simulink library "mbd_s32k1xx_ec_toolbox"  (Simulink 9.0)
settings: Solver=FixedStepDiscrete  StartTime=0.0  StopTime=10.0  FixedStep=0.1  RelTol=1e-3  EnableMultiTasking=on
InitFcn:
  | mbd_s32k_consistency_checks(bdroot(gcs));
(part 5 of 8)

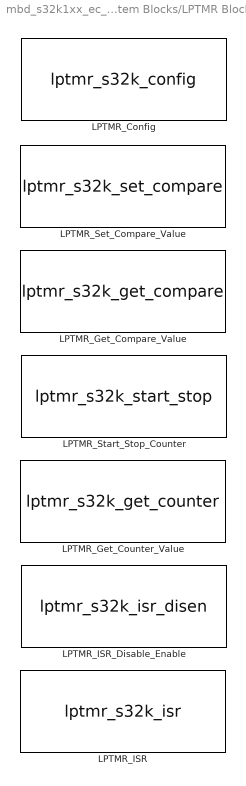
== system mbd_s32k1xx_ec_toolbox/Core and System Blocks/LPTMR Blocks ==
  LPTMR_Config : S-Function  FunctionName=lptmr_s32k_config  SFunctionDeploymentMode=off  EnableBusSupport=off  mask(lptmr_s32k_config){work_mode=Time Counter mode, compare_value=1, compare_value_units=Ticks, pin_select=Count pulses from pin alternative 1, pin_polarity=Count pulse on rising edge, pin_trgmux_source=Trigger MUX input 1, pin_gpio=PTE11: [LPTMR0_ALT1 | Low Power Timer Input Channel], show_adv_opts=on, input_clock=SIRC DIV2 clock, prescaler=Timer mode: prescaler 2, Glitch filter mode: invalid, bypass_prescaler=off, free_run=off, start_counter=on, enable_isr=off}
      mask prompts: work_mode "Mode Select"; compare_value "Compare Value"; compare_value_units "Compare Value Units"; pin_select "Pin Source"; pin_polarity "Pin Polarity"; pin_trgmux_source "TRGMUX Source"; pin_gpio "Input Pin"; show_adv_opts "Show advanced options"; input_clock "Prescaler Clock Select"; prescaler "Prescale Value"; bypass_prescaler "Prescaler Bypass"; free_run "Timer Free-Running Counter"; start_counter "Start  LPTMR counter immediatly after initialization"; enable_isr "Enable ISR immediatly after initialization"
      mask help: This block allows the user to configure the LPTMR module.
      mask init:
      | [maskStr, labels] = mbd_s32k_lptmr_init();
      | 
      | set_param(gcb, 'MaskDisplay', labels);
      settings: NameChangeFcn=mbd_s32k_name_check(gcb);
      mask Help: web(fullfile(mbd_s32k_block_help, 'lptmr', 'lptmr_config.html'));
      mask TypeOptions work_mode: Time Counter mode | Pulse Counter mode
      mask Callback work_mode:
      | mbd_s32k_lptmr_config_cbk('mode')
      | mbd_s32k_lptmr_config_cbk('pin')
      mask TypeOptions compare_value_units: Ticks | Microseconds
      mask Callback compare_value_units: mbd_s32k_lptmr_config_cbk('units')
      mask TypeOptions pin_select: Count pulses from pin alternative 1 | Count pulses from pin alternative 2 | Count pulses from pin alternative 3 | Count pulses from TRGMUX trigger
      mask Callback pin_select:
      | mbd_s32k_lptmr_config_cbk('trgmux');
      | mbd_s32k_lptmr_config_cbk('pin');
      mask TypeOptions pin_polarity: Count pulse on rising edge | Count pulse on falling edge
      mask TypeOptions pin_trgmux_source: Trigger function is disabled | Trigger MUX input 0 | Trigger MUX input 1 | Trigger MUX input 2 | Trigger MUX input 3 | Trigger MUX input 4 | Trigger MUX input 5 | Trigger MUX input 6 | Trigger MUX input 7 | Trigger MUX input 8 | Trigger MUX input 9 | Trigger MUX input 10 | Trigger MUX input 11 | CMP0 Output | LPIT Channel 0 | LPIT Channel 1 | LPIT Channel 2 | LPIT Channel 3 | LPTMR0 Trigger | FTM0 Initialize Trigger | FTM0 External Trigger | FTM1 Initialize Trigger | FTM1 External Trigger | FTM2 Initialize Trigger | FTM2 External Trigger | FTM3 Initialize Trigger | FTM3 External Trigger | ADC0_COCOA | ADC0_COCOB | ADC1_COCOA | ADC1_COCOB | PDB0 Channel 0 Trigger | PDB0 Pulse out | PDB1 Channel 0 Trigger | PDB1 Pulse out | RTC Alarm | RTC Seconds Counter | Flex IO Trigger 0 | Flex IO Trigger 1 | Flex IO Trigger 2 | Flex IO Trigger 3 | LPUART0 RX Data | LPUART0 TX Data | LPUART0 RX Idle | LPUART1 RX Data | LPUART1 TX Data | LPUART1 RX Idle | LPI2C0 Master Stop | LPI2C0 Slave Stop | LPI2C1 Master Stop | LPI2C1 Slave Stop | LPSPI0 Frame | LPSPI0 RX Data | LPSPI1 Frame | LPSPI1 RX Data | SIM Software Trigger
      mask Callback pin_trgmux_source: mbd_s32k_lptmr_config_cbk('pin');
      mask TypeOptions pin_gpio: PTE11: [LPTMR0_ALT1 | Low Power Timer Input Channel]
      mask Callback show_adv_opts: mbd_s32k_lptmr_config_cbk('show_adv_opts')
      mask TypeOptions input_clock: SIRC DIV2 clock | 1kHz LPO clock | RTC clock | PCC configured clock
      mask TypeOptions prescaler: Timer mode: prescaler 2, Glitch filter mode: invalid | Timer mode: prescaler 4, Glitch filter mode: 2 clocks | Timer mode: prescaler 8, Glitch filter mode: 4 clocks | Timer mode: prescaler 16, Glitch filter mode: 8 clocks | Timer mode: prescaler 32, Glitch filter mode: 16 clocks | Timer mode: prescaler 64, Glitch filter mode: 32 clocks | Timer mode: prescaler 128, Glitch filter mode: 64 clocks | Timer mode: prescaler 256, Glitch filter mode: 128 clocks | Timer mode: prescaler 512, Glitch filter mode: 256 clocks | Timer mode: prescaler 1024, Glitch filter mode: 512 clocks | Timer mode: prescaler 2048, Glitch filter mode: 1024 clocks | Timer mode: prescaler 4096, Glitch filter mode: 2048 clocks | Timer mode: prescaler 8192, Glitch filter mode: 4096 clocks | Timer mode: prescaler 16384, Glitch filter mode: 8192 clocks | Timer mode: prescaler 32768, Glitch filter mode: 16384 clocks | Timer mode: prescaler 65536, Glitch filter mode: 32768 clocks
      mask Callback bypass_prescaler: mbd_s32k_lptmr_config_cbk('prescaler')
      mask DialogControl timer_config_group Prompt: Timer configuration
      mask DialogControl source_config_group Prompt: Source configuration
      mask DialogControl prescaler_config_group Prompt: Prescaler configuration
      mask Display:
      | image('nxp_logo.png', 'top-right');
      | disp(maskStr);
  LPTMR_Get_Compare_Value : S-Function  FunctionName=lptmr_s32k_get_compare  Parameters=sFuncParams  SFunctionDeploymentMode=off  EnableBusSupport=off  mask(lptmr_s32k_get_compare){compare_value_units=Ticks}
      mask prompts: compare_value_units "Compare Value Units"
      mask help: This block allows the user to get the compare value in counter tick units or microseconds, for LPTMR.
      mask init:
      | [maskStr, labels, sFuncParams] = mbd_s32k_lptmr_get_compare();
      | 
      | set_param(gcb, 'MaskDisplay', labels);
      settings: NameChangeFcn=mbd_s32k_name_check(gcb);
      mask Help: web(fullfile(mbd_s32k_block_help, 'lptmr', 'lptmr_get_compare.html'));
      mask TypeOptions compare_value_units: Ticks | Microseconds
      mask Display:
      | image('nxp_logo.png', 'top-right');
      | port_label('output', 1, 'Compare Value');
      | disp(maskStr);
  LPTMR_Get_Counter_Value : S-Function  FunctionName=lptmr_s32k_get_counter  SFunctionDeploymentMode=off  EnableBusSupport=off  mask(lptmr_s32k_get_counter){}
      mask help: This block allows the user to get the current counter value in counter ticks units, for LPTMR.
      mask init:
      | [maskStr labels] = mbd_s32k_lptmr_get_counter();
      | 
      | set_param(gcb, 'MaskDisplay', labels);
      settings: NameChangeFcn=mbd_s32k_name_check(gcb);
      mask Help: web(fullfile(mbd_s32k_block_help, 'lptmr', 'lptmr_get_counter.html'));
      mask Display:
      | image('nxp_logo.png', 'top-right');
      | port_label('output', 1, 'Counter Value')
      | disp(maskStr);
  LPTMR_ISR : S-Function  FunctionName=lptmr_s32k_isr  SFunctionDeploymentMode=off  EnableBusSupport=off  mask(lptmr_s32k_isr){}
      mask help: This block allows to call user function on LPTMR interrupt.
      settings: NameChangeFcn=mbd_s32k_name_check(gcb);
      mask Help: web(fullfile(mbd_s32k_block_help, 'lptmr', 'lptmr_isr.html'));
      mask Display:
      | image('nxp_logo.png', 'top-right');
      | disp('LPTMR ISR');
  LPTMR_ISR_Disable_Enable : S-Function  FunctionName=lptmr_s32k_isr_disen  SFunctionDeploymentMode=off  EnableBusSupport=off  mask(lptmr_s32k_isr_disen){set_action=Enable}
      mask prompts: set_action "Action"
      mask help: This block allows the user to enable or disable the LPTMR.
      mask init:
      | [maskStr, labels] = mbd_s32k_lptmr_isr_disen();
      | 
      | set_param(gcb, 'MaskDisplay', labels);
      settings: NameChangeFcn=mbd_s32k_name_check(gcb);
      mask Help: web(fullfile(mbd_s32k_block_help, 'lptmr', 'lptmr_isr_disable_enable.html'));
      mask TypeOptions set_action: Enable | Disable
      mask Display:
      | image('nxp_logo.png', 'top-right');
      | disp(maskStr);
  LPTMR_Set_Compare_Value : S-Function  FunctionName=lptmr_s32k_set_compare  Parameters=sFuncParams  SFunctionDeploymentMode=off  EnableBusSupport=off  mask(lptmr_s32k_set_compare){compare_value_units=Microseconds}
      mask prompts: compare_value_units "Compare Value Units"
      mask help: This block allows the user to set the compare value in counter tick units or microsenconds, for LPTMR.
      mask init:
      | [maskStr, labels, sFuncParams] = mbd_s32k_lptmr_set_compare();
      | 
      | set_param(gcb, 'MaskDisplay', labels);
      settings: NameChangeFcn=mbd_s32k_name_check(gcb);
      mask Help: web(fullfile(mbd_s32k_block_help, 'lptmr', 'lptmr_set_compare.html'));
      mask TypeOptions compare_value_units: Ticks | Microseconds
      mask Display:
      | image('nxp_logo.png', 'top-right');
      | port_label('input', 1, 'Compare Value');
      | disp(maskStr);
  LPTMR_Start_Stop_Counter : S-Function  FunctionName=lptmr_s32k_start_stop  SFunctionDeploymentMode=off  EnableBusSupport=off  mask(lptmr_s32k_start_stop){set_action=Start}
      mask prompts: set_action "Action"
      mask help: This block allows the user to start or stop the LPTMR.
      mask init:
      | [maskStr, labels] = mbd_s32k_lptmr_start_stop();
      | 
      | set_param(gcb, 'MaskDisplay', labels);
      settings: NameChangeFcn=mbd_s32k_name_check(gcb);
      mask Help: web(fullfile(mbd_s32k_block_help, 'lptmr', 'lptmr_start_stop.html'));
      mask TypeOptions set_action: Start | Stop
      mask Display:
      | image('nxp_logo.png', 'top-right');
      | disp(maskStr);

== system mbd_s32k1xx_ec_toolbox/Core and System Blocks/PMC Blocks ==
  PMC_Config : S-Function  FunctionName=pmc_s32k_config  Parameters=sFuncParams  SFunctionDeploymentMode=off  EnableBusSupport=off  mask(pmc_s32k_config){power_mode=Very Low Power Stop (VLPS), sleep_on_exit=off, callback_before=off, callback_after=off, callback_before_after=off, show_adv_opts=off}
      mask prompts: power_mode "Power Mode"; sleep_on_exit "Sleep on exit from ISR"; callback_before "Execute subsystem "Before" entering in selected Power Mode"; callback_after "Execute subsystem "After" exiting from selected Power Mode"; callback_before_after "Execute subsystem "Before and After" selected Power Mode"; show_adv_opts "Show advanced options"
      mask help: This block allows the user to handle the device power modes and trigger subsystems execution at run-time switching between power modes.
      mask init:
      | mbd_s32k_pmc_config_cbk(gcb);
      | 
      | [st,labels] = mbd_s32k_pmc_init(gcb);
      | 
      | set_param(gcb, 'MaskDisplay', labels);
      | 
      | sFuncParams = [callback_before
      |                 callback_after
      |                 callback_before_after]';
      settings: NameChangeFcn=mbd_s32k_name_check(gcb);
      mask Help: web(fullfile(mbd_s32k_block_help, 'pmc', 'pmc_config.html'));
      mask TypeOptions power_mode: Very Low Power Stop (VLPS) | Very Low Power Run (VLPR) | High Speed Run (HSRUN) | Normal Operating (RUN) | Stop System and Bus clocks (STOP1) | Stop System clock and keep Bus clock running (STOP2)
      mask Callback power_mode: mbd_s32k_pmc_config_cbk(gcb);
      mask Callback show_adv_opts: mbd_s32k_pmc_config_cbk(gcb);
      mask DialogControl Control2 Prompt: %<MaskDescription>)
      mask DialogControl container_mode Prompt: General
      mask DialogControl Container20 Prompt: Run/Stop
      mask DialogControl container_callbacks Prompt: Callbacks
      mask Display:
      | image('nxp_logo.png', 'top-right');
      | disp(st);

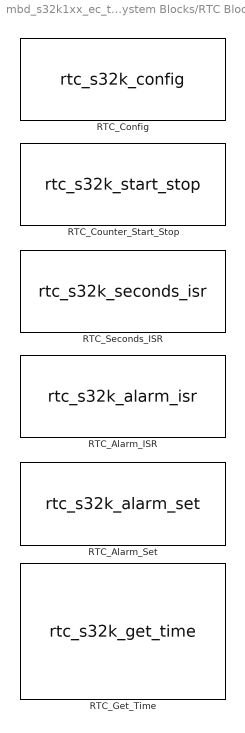
== system mbd_s32k1xx_ec_toolbox/Core and System Blocks/RTC Blocks ==
  RTC_Alarm_ISR : S-Function  FunctionName=rtc_s32k_alarm_isr  SFunctionDeploymentMode=off  EnableBusSupport=off  mask(rtc_s32k_alarm_isr){}
      mask help: This block allows to call user function on RTC interrupt.
      settings: NameChangeFcn=mbd_s32k_name_check(gcb);
      mask Help: web(fullfile(mbd_s32k_block_help, 'rtc', 'rtc_alarm_isr.html'));
      mask Display:
      | image('nxp_logo.png', 'top-right');
      | disp('RTC Alarm ISR');
  RTC_Alarm_Set : S-Function  FunctionName=rtc_s32k_alarm_set  Parameters=sFuncParams  SFunctionDeploymentMode=off  EnableBusSupport=off  mask(rtc_s32k_alarm_set){inputs_enable=on, date_day=1, date_month=1, date_year=1970, time_hour=0, time_min=0, time_sec=0, show_adv_opts=off, repeat=off, interval=0, forever=on, repeats=0}
      mask prompts: inputs_enable "Date/Time as inputs"; date_day "Date (dd/mm/yy)"; time_hour "Time (hh:mm::ss)"; show_adv_opts "Show advanced options"; interval "Repeat interval (seconds)"; forever "Repeat forever"; repeats "Number of repeats"
      mask help: This block allows the user to set an alarm.
      mask init:
      | [st, labels] = mbd_s32k_rtc_alarm_set_init();
      | sFuncParams = [inputs_enable]';
      | set_param(gcb, 'MaskDisplay', labels);
      settings: NameChangeFcn=mbd_s32k_name_check(gcb);
      mask Help: web(fullfile(mbd_s32k_block_help, 'rtc', 'rtc_alarm_set.html'));
      mask Callback inputs_enable: mbd_s32k_rtc_alarm_set_cbk('inputs_enable')
      mask Callback show_adv_opts: mbd_s32k_rtc_alarm_set_cbk('show_adv_opts')
      mask Callback repeat: mbd_s32k_rtc_alarm_set_cbk('repeat_enable')
      mask Callback forever: mbd_s32k_rtc_alarm_set_cbk('repeat_forever')
      mask Display:
      | image('nxp_logo.png', 'top-right');
      | port_label('input', 1, 'Year')
      | port_label('input', 2, 'Month')
      | port_label('input', 3, 'Day')
      | port_label('input', 4, 'Hours')
      | port_label('input', 5, 'Minutes')
      | port_label('input', 6, 'Seconds')
      | disp(st);
  RTC_Config : S-Function  FunctionName=rtc_s32k_config  SFunctionDeploymentMode=off  EnableBusSupport=off  mask(rtc_s32k_config){date_day=1, date_month=1, date_year=1970, time_hour=0, time_min=0, time_sec=0, show_adv_opts=off, clock_input=1KHz LPO, clock_output=Disabled, comp_state=on, comp_value=0, comp_interval=0, state_update=off, state_w_access=off, state_read_only=off, start_counter=on}
      mask prompts: date_day "Date"; time_hour "Time"; show_adv_opts "Show advanced options"; clock_input "Input Clock"; clock_output "Clock Out"; comp_state "Compensation"; comp_value "Compensation value            [-127,128]"; comp_interval "Compensation interval              [0,255]"; state_update "Update"; state_w_access "Non-supervisor write access"; state_read_only "Read-only"; start_counter "Start RTC counter immediatly after initialization"
      mask help: This block allows the user to configure the RTC module.
      mask init:
      | [labels ,maskStr] = mbd_s32k_rtc_config_init();
      | 
      | set_param(gcb, 'MaskDisplay', [labels, newline, 'disp(maskStr);']);
      settings: NameChangeFcn=mbd_s32k_name_check(gcb);
      mask Help: web(fullfile(mbd_s32k_block_help, 'rtc', 'rtc_config.html'));
      mask Callback show_adv_opts: mbd_s32k_rtc_config_cbk('show_adv_opts')
      mask TypeOptions clock_input: 32KHz crystal | 1KHz LPO
      mask TypeOptions clock_output: Disabled | Prescaler output | 32KHz clock
      mask Callback comp_state: mbd_s32k_rtc_config_cbk('compensation')
      mask Callback comp_interval: mbd_s32k_rtc_config_cbk('comp_value')
      mask DialogControl time_config_group Prompt: Time configuration
      mask DialogControl time_config_group_copy Prompt: Time configuration
      mask Display:
      | image('nxp_logo.png', 'top-right');
      | 
      | disp(maskStr);
  RTC_Counter_Start_Stop : S-Function  FunctionName=rtc_s32k_start_stop  SFunctionDeploymentMode=off  EnableBusSupport=off  mask(rtc_s32k_counter_start_stop){set_action=Start}
      mask prompts: set_action "Action"
      mask help: This block allows the user to start or stop the RTC counter.
      mask init:
      | [labels, maskStr] = mbd_s32k_rtc_start_stop();
      | 
      | set_param(gcb, 'MaskDisplay', [labels, 'disp(maskStr);']);
      settings: NameChangeFcn=mbd_s32k_name_check(gcb);
      mask Help: web(fullfile(mbd_s32k_block_help, 'rtc', 'rtc_counter_start_stop.html'));
      mask TypeOptions set_action: Start | Stop
      mask Display:
      | image('nxp_logo.png', 'top-right');
      | disp(maskStr);
  RTC_Get_Time : S-Function  FunctionName=rtc_s32k_get_time  SFunctionDeploymentMode=off  EnableBusSupport=off  mask(rtc_s32k_get_time){}
      mask help: This block returns the time to the user.
      mask init:
      | [st,labels] = mbd_s32k_rtc_get_time_init();
      | set_param(gcb, 'MaskDisplay', labels);
      settings: NameChangeFcn=mbd_s32k_name_check(gcb);
      mask Help: web(fullfile(mbd_s32k_block_help, 'rtc', 'rtc_get_time.html'));
      mask Display:
      | image('nxp_logo.png', 'top-right');
      | port_label('output', 1, 'Year')
      | port_label('output', 2, 'Month')
      | port_label('output', 3, 'Day')
      | port_label('output', 4, 'Hours')
      | port_label('output', 5, 'Minutes')
      | port_label('output', 6, 'Seconds')
      | disp(st);
  RTC_Seconds_ISR : S-Function  FunctionName=rtc_s32k_seconds_isr  SFunctionDeploymentMode=off  EnableBusSupport=off  mask(rtc_s32k_seconds_isr){sec_irq_freq=1Hz}
      mask prompts: sec_irq_freq "Frequency"
      mask help: This block allows to call user function on RTC interrupt.
      mask init:
      | [labels, maskStr] = mbd_s32k_rtc_seconds_isr_init();
      | 
      | set_param(gcb, 'MaskDisplay', [labels, 'disp(maskStr);']);
      settings: NameChangeFcn=mbd_s32k_name_check(gcb);
      mask Help: web(fullfile(mbd_s32k_block_help, 'rtc', 'rtc_seconds_isr.html'));
      mask TypeOptions sec_irq_freq: 1Hz | 2Hz | 4Hz | 8Hz | 16Hz | 32Hz | 64Hz | 128Hz
      mask DialogControl Container3 Prompt: General
      mask Display:
      | image('nxp_logo.png', 'top-right');
      | disp(maskStr);

== system mbd_s32k1xx_ec_toolbox/Core and System Blocks/WDOG Blocks ==
  WDOG_Config : S-Function  FunctionName=wdog_s32k_config  Parameters=sFuncParams  SFunctionDeploymentMode=off  EnableBusSupport=off  mask(wdog_s32k_config){clk_source=LPO clock, window_enable=off, window_value=1000.000, window_value_unit=milliseconds, timeout_value=1000.000, timeout_value_unit=milliseconds, prescaler_enable=on, update_enable=off, int_enable=off, show_adv_opts=off}
      mask prompts: clk_source "Clock source"; window_enable "Window enable"; window_value "Window value"; timeout_value "Timeout value"; prescaler_enable "Prescaler enable"; update_enable "Update enable"; int_enable "Interrupt enable"; show_adv_opts "Show advanced options"
      mask help: This block allows the user to configure the WDOG module.
      mask init:
      | maskStr = ['WDOG Config Block', newline, newline, ...
      |     'Clock source: ', get_param(gcb, 'clk_source')];
      | 
      | 
      | if strcmp(get_param(gcb, 'window_enable'), 'on')
      |     maskStr = [maskStr, newline];
      |     maskStr = [maskStr, 'Window: ', ...
      |         get_param(gcb, 'window_value'), ' ', ...
      |         get_param(gcb, 'window_value_unit')];
      | end
      | 
      | 
      | sFuncParams = [
      |     clk_source
      |     update_enable
      |     int_enable
      |     window_enable
      |     window_value
      |     window_value_unit
      |     timeout_value
      |     timeout_value_unit
      |     prescaler_enable];
      settings: NameChangeFcn=mbd_s32k_name_check(gcb);
      mask Help: web(fullfile(mbd_s32k_block_help, 'wdog', 'wdog_config.html'));
      mask TypeOptions clk_source: Bus clock | LPO clock | SOSC clock | SIRC clock
      mask Callback clk_source: mbd_s32k_wdog_config_cbk('clk_source')
      mask Callback window_enable: mbd_s32k_wdog_config_cbk('window_enable')
      mask Callback window_value: mbd_s32k_wdog_config_cbk('window_value')
      mask TypeOptions window_value_unit: seconds | milliseconds | microseconds | clock cycles
      mask Callback window_value_unit: mbd_s32k_wdog_config_cbk('window_value_unit')
      mask Callback timeout_value: mbd_s32k_wdog_config_cbk('timeout_value')
      mask TypeOptions timeout_value_unit: seconds | milliseconds | microseconds | clock cycles
      mask Callback timeout_value_unit: mbd_s32k_wdog_config_cbk('timeout_value_unit')
      mask Callback prescaler_enable: mbd_s32k_wdog_config_cbk('prescaler_enable')
      mask Callback show_adv_opts: mbd_s32k_wdog_config_cbk('show_adv_opts')
      mask DialogControl GeneralTab Prompt: General
      mask DialogControl SourceClockFreqText Prompt: Source clock frequency: 128 KHz
      mask DialogControl WindowGroupbox Prompt: Window
      mask DialogControl TimeoutGroupbox Prompt: Timeout
      mask Display:
      | image('nxp_logo.png', 'top-right');
      | disp(maskStr);
  WDOG_ISR : S-Function  FunctionName=wdog_s32k_isr  SFunctionDeploymentMode=off  EnableBusSupport=off  mask(wdog_s32k_isr){}
      mask help: This block allows to call user function on WDOG timeout interrupt.
      settings: NameChangeFcn=mbd_s32k_name_check(gcb);
      mask Help: web(fullfile(mbd_s32k_block_help, 'wdog', 'wdog_isr.html'));
      mask Display:
      | image('nxp_logo.png', 'top-right');
      | disp('WDOG ISR Block');
  WDOG_Trigger : S-Function  FunctionName=wdog_s32k_trigger  SFunctionDeploymentMode=off  EnableBusSupport=off  mask(wdog_s32k_trigger){}
      mask help: This block allows the user to refresh the WDOG counter.
      settings: NameChangeFcn=mbd_s32k_name_check(gcb);
      mask Help: web(fullfile(mbd_s32k_block_help, 'wdog', 'wdog_trigger.html'));
      mask Display:
      | image('nxp_logo.png', 'top-right');
      | disp('WDOG Trigger Block');

== system mbd_s32k1xx_ec_toolbox/Motor Control Blocks/ADC Blocks ==
  ADC_Config : S-Function  FunctionName=adc_s32k_config  SFunctionDeploymentMode=off  EnableBusSupport=off  mask(adc_s32k_config_block){instance=0, mode=8-bit conversion, smplts=2, adiclk=alternate clock 1, adiv=input clock, show_adv_opts=off, pretrgsel=PDB pre-trigger, swpretrg=Disabled, adtrg=software, trgsel=TRGMUX output, refsel=Vrefh and Vrefl, supply_monitoring=off, acfe=off, acfgt=off, acren=off, cv1=0, cv2=0, adco=off, avge=off, avgs=4 samples}
      mask prompts: instance "ADC"; mode "Conversion Mode Selection"; smplts "Sample Time Select (2 - 256)"; adiclk "Input Clock Select"; adiv "Clock Divide Select"; show_adv_opts "Show advanced options"; pretrgsel "Pre-trigger Source Select"; swpretrg "Software Pre-trigger Source"; adtrg "Conversion Trigger Select"; trgsel "Trigger Source"; refsel "Voltage Reference Selection"; supply_monitoring "Supply Monitoring Enable"; acfe "Compare Function Enable"; acfgt "Compare Function Greater Than Enable"; acren "Compare Function Range Enable"; cv1 "Compare Value Register 1 (0 - 65535)"; cv2 "Compare Value Register 2 (0 - 65535)"; adco "Continuous Conversion Enable"; avge "Hardware Average Enable"; avgs "Hardware Average Select"
      mask help: This block allows the user to configure the ADC module
      mask init:
      | maskStr = mbd_s32k_adc_config_init();
      settings: NameChangeFcn=mbd_s32k_name_check(gcb);
      mask Help: web(fullfile(mbd_s32k_block_help, 'adc', 'adc_config_block.html'));
      mask TypeOptions instance: 0 | 1
      mask Callback instance: mbd_s32k_adc_display_instances();
      mask TypeOptions mode: 8-bit conversion | 10-bit conversion | 12-bit conversion
      mask Callback smplts:
      | s = get_param(gcb, 'smplts');
      | s = str2num(s);
      | if isempty(s), s = 0; end
      | if s < 2, s = 2; end
      | if s > 256, s = 256; end
      | set_param(gcb, 'smplts', num2str(s));
      | clear s
      mask TypeOptions adiclk: alternate clock 1
      mask TypeOptions adiv: input clock | input clock / 2 | input clock / 4 | input clock / 8
      mask Callback show_adv_opts: mbd_s32k_adc_config_cbk('show_adv_opts');
      mask TypeOptions pretrgsel: PDB pre-trigger | TRGMUX pre-trigger | Software pre-trigger
      mask Callback pretrgsel: mbd_s32k_adc_config_cbk('pretrgsel');
      mask TypeOptions swpretrg: Disabled | Software pre-trigger 0 | Software pre-trigger 1 | Software pre-trigger 2 | Software pre-trigger 3
      mask TypeOptions adtrg: software | hardware
      mask Callback adtrg: mbd_s32k_adc_config_cbk('adtrg');
      mask TypeOptions trgsel: PDB output | TRGMUX output
      mask TypeOptions refsel: Vrefh and Vrefl | Valth and Valtl
      mask Callback acfe: mbd_s32k_adc_config_cbk('acfe');
      mask Callback acren: mbd_s32k_adc_config_cbk('acren');
      mask Callback cv1:
      | value = str2num(get_param(gcb, 'cv1'));
      | if isempty(value), value = 0; end
      | if (value > 65535)
      |     value = 65535;
      | elseif (value < 0)
      |     value = 0;
      | end
      | set_param(gcb, 'cv1', num2str(value));
      mask Callback cv2:
      | value = str2num(get_param(gcb, 'cv2'));
      | if isempty(value), value = 0; end
      | if (value > 65535)
      |     value = 65535;
      | elseif (value < 0)
      |     value = 0;
      | end
      | set_param(gcb, 'cv2', num2str(value));
      mask Callback avge: mbd_s32k_adc_config_cbk('avge');
      mask TypeOptions avgs: 4 samples | 8 samples | 16 samples | 32 samples
      mask DialogControl ParameterGroupVar0 Prompt: Clock Configuration
      mask DialogControl ParameterGroupVar01 Prompt: Compare Configuration
      mask DialogControl ParameterGroupVar012 Prompt: Conversion Configuration
      mask Display:
      | image('nxp_logo.png', 'top-right');
      | disp(maskStr);
  ADC_ISR : S-Function  FunctionName=adc_s32k_isr  SFunctionDeploymentMode=off  EnableBusSupport=off  mask(adc_s32k_isr_block){instance=0, pri=0, sc1n=A}
      mask prompts: instance "ADC"; pri "Interrupt Priority"; sc1n "SC1 Register"
      mask help: This block allows triggering of a subsystem on ADC conversion events and getting the conversion results, as well as the channel.
      mask init:
      | maskStr = mbd_s32k_adc_isr_string();
      settings: NameChangeFcn=mbd_s32k_name_check(gcb);
      mask Help: web(fullfile(mbd_s32k_block_help, 'adc', 'adc_isr_block.html'));
      mask TypeOptions instance: 0 | 1
      mask Callback instance: mbd_s32k_adc_display_instances();
      mask TypeOptions pri: 0 | 1 | 2 | 3 | 4 | 5 | 6 | 7 | 8 | 9 | 10 | 11 | 12 | 13 | 14 | 15
      mask Callback pri: mbd_s32k_isr_priority_cbk(gcb, 'pri');
      mask TypeOptions sc1n: A | B | C | D | E | F | G | H | I | J | K | L | M | N | O | P
      mask Display:
      | image('nxp_logo.png', 'top-right');
      | disp(maskStr);
      | port_label('output',1,'function')
      | port_label('output',2,'data result')
      | port_label('output',3,'channel')
  ADC_Interleave : S-Function  FunctionName=adc_s32k_interleave  SFunctionDeploymentMode=off  EnableBusSupport=off  mask(adc_s32k_interleave_block){adcInterleavePins=PTB0 to ADC0_SE4 and ADC1_SE14, adcInterleaveInit=on}
      mask prompts: adcInterleavePins "Select ADC interleave pins"; adcInterleaveInit "Place the code in initialization function"
      mask help: ADC interleave channel enable
      mask init:
      | [maskStr] = mbd_s32k_adc_interleave_init();
      mask Help: web(fullfile(mbd_s32k_block_help, 'adc', 'adc_interleave_block.html'));
      mask TypeOptions adcInterleavePins: PTB0 to ADC0_SE4 and ADC1_SE14 | PTB1 to ADC0_SE5 and ADC1_SE15 | PTB13 to ADC1_SE8 and ADC0_SE8 | PTB14 to ADC1_SE9 and ADC0_SE9
      mask Callback adcInterleavePins: mbd_s32k_adc_interleave_cbk()
      mask Display:
      | image('nxp_logo.png', 'top-right');
      | disp(maskStr);
  ADC_Start : S-Function  FunctionName=adc_s32k_start  Parameters=out  SFunctionDeploymentMode=off  EnableBusSupport=off  mask(adc_s32k_start_block){instance=0, adc_r=A, adc_chan=PTA0: [ADC0_SE0 | ADC Single Ended Input], aien=off, mcuTargetUpdate=on}
      mask prompts: instance "ADC"; adc_r "SC1 Register"; adc_chan "Input Channel"; aien "Interrupt Enable"
      mask help: This block allows to configure channel parameters, start the conversion and get the result when interrupt is not enabled.
      mask init:
      | [maskStr, out] = mbd_s32k_adc_start_string();
      | mbd_s32k_adc_start_display();
      settings: NameChangeFcn=mbd_s32k_name_check(gcb);
      mask Help: web(fullfile(mbd_s32k_block_help, 'adc', 'adc_start_block.html'));
      mask TypeOptions instance: 0 | 1
      mask Callback instance:
      | mbd_s32k_adc_start_display();
      | mbd_s32k_adc_display_instances();
      mask TypeOptions adc_r: A | B | C | D | E | F | G | H | I | J | K | L | M | N | O | P
      mask TypeOptions adc_chan: PTA0: [ADC0_SE0 | ADC Single Ended Input] | PTA1: [ADC0_SE1 | ADC Single Ended Input] | PTA6: [ADC0_SE2 | ADC Single Ended Input] | PTA7: [ADC0_SE3 | ADC Single Ended Input] | PTB0: [ADC0_SE4 | ADC Single Ended Input] | PTB1: [ADC0_SE5 | ADC Single Ended Input] | PTB2: [ADC0_SE6 | ADC Single Ended Input] | PTB3: [ADC0_SE7 | ADC Single Ended Input] | PTB13: [ADC0_SE8 | ADC Single Ended Input] | PTC0: [ADC0_SE8 | ADC Single Ended Input] | PTB14: [ADC0_SE9 | ADC Single Ended Input] | PTC1: [ADC0_SE9 | ADC Single Ended Input] | PTC2: [ADC0_SE10 | ADC Single Ended Input] | PTC3: [ADC0_SE11 | ADC Single Ended Input] | PTC14: [ADC0_SE12 | ADC Single Ended Input] | PTC15: [ADC0_SE13 | ADC Single Ended Input] | PTC16: [ADC0_SE14 | ADC Single Ended Input] | PTC17: [ADC0_SE15 | ADC Single Ended Input] | PTB18: [ADC0_SE16 | ADC Single Ended Input] | PTB20: [ADC0_SE17 | ADC Single Ended Input] | PTB21: [ADC0_SE18 | ADC Single Ended Input] | PTB22: [ADC0_SE19 | ADC Single Ended Input] | PTB23: [ADC0_SE20 | ADC Single Ended Input] | PTB25: [ADC0_SE21 | ADC Single Ended Input] | PTB27: [ADC0_SE22 | ADC Single Ended Input] | PTB28: [ADC0_SE23 | ADC Single Ended Input] | PTB29: [ADC0_SE24 | ADC Single Ended Input] | PTC19: [ADC0_SE25 | ADC Single Ended Input] | PTC23: [ADC0_SE26 | ADC Single Ended Input] | PTC27: [ADC0_SE27 | ADC Single Ended Input] | PTC28: [ADC0_SE28 | ADC Single Ended Input] | PTC29: [ADC0_SE29 | ADC Single Ended Input] | PTC30: [ADC0_SE30 | ADC Single Ended Input] | PTC31: [ADC0_SE31 | ADC Single Ended Input] | Temp Sensor | Band Gap | VREFSH | VREFSL | Module is disabled | VDD | VDDA | VREFH | VDD 3V | VDD FLASH 3V | VDD LV
      mask Callback adc_chan: mbd_s32k_adc_start_display();
      mask DialogControl ParameterTabVar0 Prompt: General
      mask Display:
      | image('nxp_logo.png', 'top-right');
      | disp(maskStr);

== system mbd_s32k1xx_ec_toolbox/Motor Control Blocks/CMP Blocks ==
  CMP_Config : S-Function  FunctionName=cmp_s32k_config  SFunctionDeploymentMode=off  EnableBusSupport=off  mask(cmp_s32k_config){instance=0, mode=Sampled Filtered Ext Clock, fpr=0, pmode=Low Speed, invt=off, cos=Set CMPO to equal COUT (filtered), ope=PTE3: [CMP0_OUT | Comparator Output trigger], filter_cnt=Disabled, offset=level 0, hystctr=level 0, inpsel=IN0, from the 8-bit DAC output, innsel=IN0, from the 8-bit DAC output, chn0=off, chn1=off, chn2=off, chn3=off, chn4=off, chn5=off, chn6=off, chn7=off, dacen=on, vrsel=Vin1, psel=PTA0: [CMP0_IN0 | Comparator Input Signal], msel=PTA1: [CMP0_IN1 | Comparator Input Signal], vosel=0, rre=off, fxmp=The Plus port is fixed, fxmxch=Channel 0, nsam=as soon as the active channel is scanned, mcuTargetUpdate=on}
      mask prompts: instance "CMP"; fpr "Filter Sample Period"; pmode "Power Mode Select"; invt "Comparator Invert"; cos "Comparator Output Select"; ope "Comparator Output Pin Enable"; filter_cnt "Filter Sample Count"; offset "Offset Control"; hystctr "Hysteresis Control"; inpsel "Selection of the input to the positive port"; innsel "Selection of the input to the negative port"; chn0 "Channel 0 input enable"; chn1 "Channel 1 input enable"; chn2 "Channel 2 input enable"; chn3 "Channel 3 input enable"; chn4 "Channel 4 input enable"; chn5 "Channel 5 input enable"; chn6 "Channel 6 input enable"; chn7 "Channel 7 input enable"; dacen "DAC Enable"; vrsel "Supply Voltage Reference Source Select"; psel "Plus Input MUX Control"; msel "Minus Input MUX Control"; vosel "DAC Output Voltage Select"; rre "Round-Robin Enable"; fxmp "Fixed MUX Port"; fxmxch "Fixed Channel Selection"; nsam "Number of Sample Clocks"
      mask help: This block allows to configure CMP module.
      mask init:
      | [maskStr] = mbd_s32k_cmp_config_init();
      | mbd_s32k_cmp_config_display;
      settings: NameChangeFcn=mbd_s32k_name_check(gcb);
      mask Help: web(fullfile(mbd_s32k_block_help, 'cmp', 'cmp_config.html'));
      mask TypeOptions instance: 0
      mask TypeOptions mode: Continuous | Sampled Non-Filtered Int Clock | Sampled Non-Filtered Ext Clock | Sampled Filtered Int Clock | Sampled Filtered Ext Clock | Window | Windowed Resampled | Windowed Filtered
      mask Callback mode: mbd_s32k_cmp_config_cbk('mode');
      mask Callback fpr: mbd_s32k_cmp_config_cbk('fpr');
      mask TypeOptions pmode: Low Speed | High Speed
      mask TypeOptions cos: Set CMPO to equal COUT (filtered) | Set CMPO to equal COUTA (unfiltered)
      mask TypeOptions ope: PTA4: [CMP0_OUT | Comparator Output trigger] | PTE3: [CMP0_OUT | Comparator Output trigger]
      mask TypeOptions filter_cnt: Disabled | 1 consecutive sample must agree | 2 consecutive samples must agree | 3 consecutive samples must agree | 4 consecutive samples must agree | 5 consecutive samples must agree | 6 consecutive samples must agree | 7 consecutive samples must agree
      mask TypeOptions offset: level 0 | level 1
      mask TypeOptions hystctr: level 0 | level 1 | level 2 | level 3
      mask TypeOptions inpsel: IN0, from the 8-bit DAC output | IN1, from the analog 8-1 mux
      mask TypeOptions innsel: IN0, from the 8-bit DAC output | IN1, from the analog 8-1 mux
      mask TypeOptions vrsel: Vin1 | Vin2
      mask TypeOptions psel: PTA0: [CMP0_IN0 | Comparator Input Signal] | PTA1: [CMP0_IN1 | Comparator Input Signal] | PTC4: [CMP0_IN2 | Comparator Input Signal] | PTE8: [CMP0_IN3 | Comparator Input Signal] | PTC3: [CMP0_IN4 | Comparator Input Signal] | PTC2: [CMP0_IN5 | Comparator Input Signal] | PTD7: [CMP0_IN6 | Comparator Input Signal] | PTD6: [CMP0_IN7 | Comparator Input Signal]
      mask TypeOptions msel: PTA0: [CMP0_IN0 | Comparator Input Signal] | PTA1: [CMP0_IN1 | Comparator Input Signal] | PTC4: [CMP0_IN2 | Comparator Input Signal] | PTE8: [CMP0_IN3 | Comparator Input Signal] | PTC3: [CMP0_IN4 | Comparator Input Signal] | PTC2: [CMP0_IN5 | Comparator Input Signal] | PTD7: [CMP0_IN6 | Comparator Input Signal] | PTD6: [CMP0_IN7 | Comparator Input Signal]
      mask Callback vosel: mbd_s32k_cmp_config_cbk('vosel');
      mask TypeOptions fxmp: The Plus port is fixed | The Minus port is fixed
      mask TypeOptions fxmxch: Channel 0 | Channel 1 | Channel 2 | Channel 3 | Channel 4 | Channel 5 | Channel 6 | Channel 7
      mask TypeOptions nsam: as soon as the active channel is scanned | 1 round-robin clock cycle after the next cycle | 2 round-robin clock cycles after the next cycle | 3 round-robin clock cycles after the next cycle
      mask Display:
      | image('nxp_logo.png', 'top-right');
      | disp(maskStr);
  CMP_ISR : S-Function  FunctionName=cmp_s32k_isr  SFunctionDeploymentMode=off  EnableBusSupport=off  mask(cmp_s32k_isr){instance=0, ier=off, ief=off, prio=0}
      mask prompts: instance "CMP"; ier "Rising ISR"; ief "Falling ISR"; prio "ISR Priority"
      mask help: This block allows to configure Comparator ISR routine.
      mask init:
      | [maskStr] = mbd_s32k_cmp_isr_init();
      settings: NameChangeFcn=mbd_s32k_name_check(gcb);
      mask Help: web(fullfile(mbd_s32k_block_help, 'cmp', 'cmp_isr.html'));
      mask TypeOptions instance: 0
      mask TypeOptions prio: 0 | 1 | 2 | 3 | 4 | 5 | 6 | 7 | 8 | 9 | 10 | 11 | 12 | 13 | 14 | 15
      mask Callback prio: mbd_s32k_isr_priority_cbk(gcb, 'prio')
      mask DialogControl ParameterTabVar0 Prompt: General
      mask Display:
      | image('nxp_logo.png', 'top-right');
      | disp(maskStr);
      | port_label('output',1,'trigger');
      | port_label('output',2,'CFR');
      | port_label('output',3,'CFF');
  CMP_ISR_Enable_Disable : S-Function  FunctionName=cmp_s32k_isr_disen  SFunctionDeploymentMode=off  EnableBusSupport=off  mask(cmp_s32k_control_isr_disen){instance=0, ier=off, ief=off}
      mask prompts: instance "CMP"; ier "Rising ISR"; ief "Falling ISR"
      mask help: This block enables or disables the interrupts for CMP block.
      mask init:
      | [maskStr] = mbd_s32k_cmp_isr_disen_init();
      settings: NameChangeFcn=mbd_s32k_name_check(gcb);
      mask Help: web(fullfile(mbd_s32k_block_help, 'cmp', 'cmp_isr_disen.html'));
      mask TypeOptions instance: 0
      mask Display:
      | image('nxp_logo.png', 'top-right');
      | disp(maskStr);
